simulink model "SpatialKineticsOffline"  (R2013a)
settings: Solver=ode4  StartTime=0.0  StopTime=tf  FixedStep=.001  RelTol=1e-3
PreLoadFcn:
  | load DarkLowerCoeffs
  | load DarkMiddleCoeffs
  | load DarkUpperCoeffs
  | load breaks
values from neighbouring files (symbols this model uses):
  alpha = [ -2.61*pcm -0.53*pcm ]    [SpatialKineticsOpenSourceMain.m]
  breaks = DarkLowerBreaks    [SpatialKineticsOpenSourceMain.m]
  BRIO = 4.266e7    (= 42660000)    [SpatialKineticsOpenSourceMain.m]
  cpc = 2414    [SpatialKineticsOpenSourceMain.m]
  cpp = 2414    [SpatialKineticsOpenSourceMain.m]
  DarkLowerCoeffs = ppDarkLower.coefs    [SpatialKineticsOpenSourceMain.m]
  DarkMiddleCoeffs = ppDarkMiddle.coefs    [SpatialKineticsOpenSourceMain.m]
  DarkRodWorthInserted = -5*Beta    (= -0.00815)    [SpatialKineticsOpenSourceMain.m]
  DarkUpperCoeffs = ppDarkUpper.coefs    [SpatialKineticsOpenSourceMain.m]
  downcomerTimeConstant = 5    [SpatialKineticsOpenSourceMain.m]
  downIO = 216.6*ones(1,3)    [SpatialKineticsOpenSourceMain.m]
  Kc1 = 1/(rho_secondary*V_secondary)    (= 0.00032726218348)    [SpatialKineticsOpenSourceMain.m]
  Kc2 = (h_secondary*A)/(cps*rho_secondary*V_secondary)    (= 1.23242359038)    [SpatialKineticsOpenSourceMain.m]
  Kh1 = 1/(rho_primary*V_primary)    (= 0.000447917898441)    [SpatialKineticsOpenSourceMain.m]
  Kh2 = (h_primary*A)/(cpp*rho_primary*V_primary)    (= 1.29038206968)    [SpatialKineticsOpenSourceMain.m]
  Kw1 = h_primary    (= 23800)    [SpatialKineticsOpenSourceMain.m]
  Kw2 = h_secondary    (= 24500)    [SpatialKineticsOpenSourceMain.m]
  Kw3 = A/(rho_tube*cpw*V_tube)    (= 0.000122049789882)    [SpatialKineticsOpenSourceMain.m]
  PHX_IO = [649.8 637.9 643.7]    [SpatialKineticsOpenSourceMain.m]
  PHX_PI_IO = 271.8    [SpatialKineticsOpenSourceMain.m]
  rate_pct = rate/100    [SpatialKineticsOfflineMain.m]
  rcp_activatetime = 20    [SpatialKineticsOpenSourceMain.m]
  rcpt = 0.1    [SpatialKineticsOpenSourceMain.m]
  reactor_PI_IO = 0.8574    [SpatialKineticsOpenSourceMain.m]
  SVIO = zeros(1,17)    [SpatialKineticsOpenSourceMain.m]
  Ts = 0.001    [SpatialKineticsOpenSourceMain.m]
  xfc0 = -Atemp\btemp*u0    [SpatialKineticsOpenSourceMain.m]
  zone1_IO = [1.041 0.01764 0.04848]    [SpatialKineticsOpenSourceMain.m]
  zone1_thermal_IO = [1044 658.3]    [SpatialKineticsOpenSourceMain.m]
  zone2_IO = [1.098 0.0186 0.05114]    [SpatialKineticsOpenSourceMain.m]
  zone2_thermal_IO = [1083 675.9]    [SpatialKineticsOpenSourceMain.m]
  zone3_IO = [0.9147 0.01549 0.04259]    [SpatialKineticsOpenSourceMain.m]
  zone3_thermal_IO = [1031 692.5]    [SpatialKineticsOpenSourceMain.m]
libraries: simulink x36
(part 3 of 5)

== system SpatialKineticsOffline/RX #2/Parasitic Heat Loss Resulting from DRACS HXs2 ==
  "T_hot " : Inport
  T_cold : Inport  Port=2
  Primary Mass Flow Rate : Inport  Port=3
  MATLAB Function : MATLAB Function  TreatAsAtomicUnit=on
  Specific heat capacity of primary coolant : Constant  Value=cpp
  Total Power Out : Outport
  Power Lost : Outport  Port=2
  Hot Leg Reduction : Outport  Port=3
  wires:
  MATLAB Function/3(Th_red) -> Hot Leg Reduction/1
  MATLAB Function/2(Ploss_MW) -> Power Lost/1
  MATLAB Function/1(P_MW) -> Total Power Out/1
  "T_hot "/1 -> MATLAB Function/1(T_hot)
  T_cold/1 -> MATLAB Function/2(T_cold)
  Primary Mass Flow Rate/1 -> MATLAB Function/3(mdoth)
  Specific heat capacity of primary coolant/1 -> MATLAB Function/4(cpp)

== system SpatialKineticsOffline/RX #2/Primary Heat Exchanger Lumped Model #4 ==
  Primary mass flow  in : Inport
  Primary temp in : Inport  Port=2
  Secondary temp in : Inport  Port=3
  Secondary mass flow in : Inport  Port=4
  Constant : Constant  Value=Kh1  SampleTime=Ts
  Constant1 : Constant  Value=Kh2  SampleTime=Ts
  Constant2 : Constant  Value=Kc1  SampleTime=Ts
  Constant3 : Constant  Value=Kc2  SampleTime=Ts
  Constant4 : Constant  Value=Kw1  SampleTime=Ts
  Constant5 : Constant  Value=Kw2  SampleTime=Ts
  Constant6 : Constant  Value=Kw3  SampleTime=Ts
  Constant7 : Constant  Value=cpp  SampleTime=Ts
  Demux : Demux  Outputs=3
  Display : Display
  Integrator : Integrator  InitialCondition=PHX_IO
  MATLAB Function : MATLAB Function  TreatAsAtomicUnit=on
  Mux2 : Mux  Inputs=7
  Product : Product
  Product1 : Product
  Sum : Sum  Inputs=|+-
  Terminator : Terminator
  W to MW : Gain  Gain=1e-6
  PHx1_Tho : Outport
  PHx1_Tco : Outport  Port=2
  PHx1_HXout : Outport  Port=3
  wires:
  Constant/1 -> Mux2/1
  Constant1/1 -> Mux2/2
  Constant2/1 -> Mux2/3
  Constant3/1 -> Mux2/4
  Constant4/1 -> Mux2/5
  Constant5/1 -> Mux2/6
  Constant6/1 -> Mux2/7
  Mux2/1 -> [PHXpar]
  MATLAB Function/1(dx) -> Integrator/1
  [PHXpar] -> MATLAB Function/6(hxpar)
  Primary temp in/1 -> [Thi], MATLAB Function/2(Thi_input)
  Secondary temp in/1 -> MATLAB Function/3(Tci_input)
  Secondary mass flow in/1 -> MATLAB Function/5(mdotc_input)
  Primary mass flow  in/1 -> [mdoth], MATLAB Function/4(mdoth_input)
  Integrator/1 -> Display/1, Demux/1, MATLAB Function/1(x)
  Demux/3 -> Terminator/1
  Demux/2 -> PHx1_Tco/1
  Demux/1 -> [Tho], PHx1_Tho/1
  Constant7/1 -> Product/2
  [mdoth] -> Product/1
  [Thi] -> Sum/1
  [Tho] -> Sum/2
  Product/1 -> Product1/1
  Sum/1 -> Product1/2
  Product1/1 -> W to MW/1
  W to MW/1 -> PHx1_HXout/1

== system SpatialKineticsOffline/RX #2/Primary Heat Exchanger Lumped Model #5 ==
  Primary mass flow  in : Inport
  Primary temp in : Inport  Port=2
  Secondary temp in : Inport  Port=3
  Secondary mass flow in : Inport  Port=4
  Constant : Constant  Value=Kh1  SampleTime=Ts
  Constant1 : Constant  Value=Kh2  SampleTime=Ts
  Constant2 : Constant  Value=Kc1  SampleTime=Ts
  Constant3 : Constant  Value=Kc2  SampleTime=Ts
  Constant4 : Constant  Value=Kw1  SampleTime=Ts
  Constant5 : Constant  Value=Kw2  SampleTime=Ts
  Constant6 : Constant  Value=Kw3  SampleTime=Ts
  Constant7 : Constant  Value=cpp  SampleTime=Ts
  Demux : Demux  Outputs=3
  Display : Display
  Integrator : Integrator  InitialCondition=PHX_IO
  MATLAB Function : MATLAB Function  TreatAsAtomicUnit=on
  Mux2 : Mux  Inputs=7
  Product : Product
  Product1 : Product
  Sum : Sum  Inputs=|+-
  Terminator : Terminator
  W to MW : Gain  Gain=1e-6
  PHx1_Tho : Outport
  PHx1_Tco : Outport  Port=2
  PHx1_HXout : Outport  Port=3
  wires:
  Constant/1 -> Mux2/1
  Constant1/1 -> Mux2/2
  Constant2/1 -> Mux2/3
  Constant3/1 -> Mux2/4
  Constant4/1 -> Mux2/5
  Constant5/1 -> Mux2/6
  Constant6/1 -> Mux2/7
  Mux2/1 -> [PHXpar]
  MATLAB Function/1(dx) -> Integrator/1
  [PHXpar] -> MATLAB Function/6(hxpar)
  Primary temp in/1 -> [Thi], MATLAB Function/2(Thi_input)
  Secondary temp in/1 -> MATLAB Function/3(Tci_input)
  Secondary mass flow in/1 -> MATLAB Function/5(mdotc_input)
  Primary mass flow  in/1 -> [mdoth], MATLAB Function/4(mdoth_input)
  Integrator/1 -> Display/1, Demux/1, MATLAB Function/1(x)
  Demux/3 -> Terminator/1
  Demux/2 -> PHx1_Tco/1
  Demux/1 -> [Tho], PHx1_Tho/1
  Constant7/1 -> Product/2
  [mdoth] -> Product/1
  [Thi] -> Sum/1
  [Tho] -> Sum/2
  Product/1 -> Product1/1
  Sum/1 -> Product1/2
  Product1/1 -> W to MW/1
  W to MW/1 -> PHx1_HXout/1

== system SpatialKineticsOffline/RX #2/Primary Heat Exchanger Lumped Model #6 ==
  Primary mass flow  in : Inport
  Primary temp in : Inport  Port=2
  Secondary temp in : Inport  Port=3
  Secondary mass flow in : Inport  Port=4
  Constant : Constant  Value=Kh1  SampleTime=Ts
  Constant1 : Constant  Value=Kh2  SampleTime=Ts
  Constant2 : Constant  Value=Kc1  SampleTime=Ts
  Constant3 : Constant  Value=Kc2  SampleTime=Ts
  Constant4 : Constant  Value=Kw1  SampleTime=Ts
  Constant5 : Constant  Value=Kw2  SampleTime=Ts
  Constant6 : Constant  Value=Kw3  SampleTime=Ts
  Constant7 : Constant  Value=cpp  SampleTime=Ts
  Demux : Demux  Outputs=3
  Display : Display
  Integrator : Integrator  InitialCondition=PHX_IO
  MATLAB Function : MATLAB Function  TreatAsAtomicUnit=on
  Mux2 : Mux  Inputs=7
  Product : Product
  Product1 : Product
  Sum : Sum  Inputs=|+-
  Terminator : Terminator
  W to MW : Gain  Gain=1e-6
  PHx1_Tho : Outport
  PHx1_Tco : Outport  Port=2
  PHx1_HXout : Outport  Port=3
  wires:
  Constant7/1 -> Product/2
  [mdoth] -> Product/1
  [Thi] -> Sum/1
  [Tho] -> Sum/2
  Product/1 -> Product1/1
  Sum/1 -> Product1/2
  Product1/1 -> W to MW/1
  W to MW/1 -> PHx1_HXout/1
  Constant/1 -> Mux2/1
  Constant1/1 -> Mux2/2
  Constant2/1 -> Mux2/3
  Constant3/1 -> Mux2/4
  Constant4/1 -> Mux2/5
  Constant5/1 -> Mux2/6
  Constant6/1 -> Mux2/7
  Mux2/1 -> [PHXpar]
  MATLAB Function/1(dx) -> Integrator/1
  [PHXpar] -> MATLAB Function/6(hxpar)
  Primary temp in/1 -> [Thi], MATLAB Function/2(Thi_input)
  Secondary temp in/1 -> MATLAB Function/3(Tci_input)
  Secondary mass flow in/1 -> MATLAB Function/5(mdotc_input)
  Primary mass flow  in/1 -> [mdoth], MATLAB Function/4(mdoth_input)
  Integrator/1 -> Display/1, Demux/1, MATLAB Function/1(x)
  Demux/3 -> Terminator/1
  Demux/2 -> PHx1_Tco/1
  Demux/1 -> [Tho], PHx1_Tho/1

== system SpatialKineticsOffline/RX #2/Ramp Power1 ==
  Max Demand : Inport
  Add : Sum
  Clock : Clock
  Ramp : simulink/Sources/Ramp  slope=rate_pct*42/60  start=tf/2  X0=-rate_pct*42/60*tf/2
  Ramp1 : simulink/Sources/Ramp  slope=-rate_pct*42/60  start=0  X0=0
  Switch : Switch  Threshold=tf/2
  Current Demand : Outport
  wires:
  Switch/1 -> Add/2
  Clock/1 -> Switch/2
  Ramp1/1 -> Switch/3
  Ramp/1 -> Switch/1
  Add/1 -> Current Demand/1
  Max Demand/1 -> Add/1

== system SpatialKineticsOffline/RX #2/Ramp Power2 ==
  Max Demand : Inport
  Add : Sum
  Clock : Clock
  Ramp : simulink/Sources/Ramp  slope=rate_pct*42/60  start=tf/2  X0=-rate_pct*42/60*tf/2
  Ramp1 : simulink/Sources/Ramp  slope=-rate_pct*42/60  start=0  X0=0
  Switch : Switch  Threshold=tf/2
  Current Demand : Outport
  wires:
  Switch/1 -> Add/2
  Clock/1 -> Switch/2
  Ramp1/1 -> Switch/3
  Ramp/1 -> Switch/1
  Add/1 -> Current Demand/1
  Max Demand/1 -> Add/1

== system SpatialKineticsOffline/RX #2/Ramp Power3 ==
  Max Demand : Inport
  Add : Sum
  Clock : Clock
  Ramp : simulink/Sources/Ramp  slope=rate_pct*42/60  start=tf/2  X0=-rate_pct*42/60*tf/2
  Ramp1 : simulink/Sources/Ramp  slope=-rate_pct*42/60  start=0  X0=0
  Switch : Switch  Threshold=tf/2
  Current Demand : Outport
  wires:
  Switch/1 -> Add/2
  Clock/1 -> Switch/2
  Ramp1/1 -> Switch/3
  Ramp/1 -> Switch/1
  Add/1 -> Current Demand/1
  Max Demand/1 -> Add/1

== system SpatialKineticsOffline/RX #2/Reactor Outlet Temperature PI Controller1 ==
  In1 : Inport
  Display : Display
  Display1 : Display
  Display2 : Display
  Gain2 : Gain  Gain=0.01
  Gain5 : Gain  Gain=100
  Integrator : Integrator  InitialCondition=reactor_PI_IO
  Kp : Gain  Gain=.01
  Saturation : Saturate  UpperLimit=1  LowerLimit=0
  Sum12 : Sum  Inputs=+-|
  Sum13 : Sum  Inputs=|+-
  Sum2 : Sum  Inputs=|++
  Out1 : Outport
  wires:
  In1/1 -> Kp/1, Sum13/1
  Sum2/1 -> Display/1, Sum12/1, Saturation/1
  Gain2/1 -> Integrator/1
  Integrator/1 -> Display2/1, Sum2/2
  Kp/1 -> Display1/1, Sum2/1
  Saturation/1 -> Sum12/2, Out1/1
  Sum12/1 -> Gain5/1
  Sum13/1 -> Gain2/1
  Gain5/1 -> Sum13/2

== system SpatialKineticsOffline/RX #2/Secondary-side RCP Dynamics #4 ==
  In1 : Inport
  Digital Clock #1 : DigitalClock  SampleTime=Ts
  RCP #1 : TransferFcn  Numerator=[rcpt]  Denominator=[1 rcpt]
  RCP Dynamics Switch #1 : Switch  Threshold=rcp_activatetime
  Out1 : Outport
  wires:
  In1/1 -> RCP #1/1, RCP Dynamics Switch #1/3
  Digital Clock #1/1 -> RCP Dynamics Switch #1/2
  RCP #1/1 -> RCP Dynamics Switch #1/1
  RCP Dynamics Switch #1/1 -> Out1/1

== system SpatialKineticsOffline/RX #2/Secondary-side RCP Dynamics #5 ==
  In1 : Inport
  Digital Clock#2 : DigitalClock  SampleTime=Ts
  RCP #2 : TransferFcn  Numerator=[rcpt]  Denominator=[1 rcpt]
  RCP Dynamics Switch #2 : Switch  Threshold=rcp_activatetime
  Out1 : Outport
  wires:
  RCP Dynamics Switch #2/1 -> Out1/1
  In1/1 -> RCP #2/1, RCP Dynamics Switch #2/3
  Digital Clock#2/1 -> RCP Dynamics Switch #2/2
  RCP #2/1 -> RCP Dynamics Switch #2/1

== system SpatialKineticsOffline/RX #2/Secondary-side RCP Dynamics #6 ==
  In1 : Inport
  Digital Clock #3 : DigitalClock  SampleTime=Ts
  RCP #3 : TransferFcn  Numerator=[rcpt]  Denominator=[1 rcpt]
  RCP Dynamics Switch #3 : Switch  Threshold=rcp_activatetime
  Out1 : Outport
  wires:
  RCP #3/1 -> RCP Dynamics Switch #3/1
  Digital Clock #3/1 -> RCP Dynamics Switch #3/2
  In1/1 -> RCP #3/1, RCP Dynamics Switch #3/3
  RCP Dynamics Switch #3/1 -> Out1/1

== system SpatialKineticsOffline/RX #3/Downcomer mixing dynamics ==
  PHX Primary Flow 1 : Inport
  PHX Primary Flow 2 : Inport  Port=2
  PHX Primary Flow 3 : Inport  Port=3
  PHX Primary Temp 1 : Inport  Port=4
  PHX Primary Temp 2 : Inport  Port=5
  PHX Primary Temp 3 : Inport  Port=6
  Constant5 : Constant  Value=[0,downcomerTimeConstant]
  Display : Display
  Integrator : Integrator  InitialCondition=downIO
  MATLAB Function1 : MATLAB Function  TreatAsAtomicUnit=on
  Primary Mass Flow Rate : Outport
  Temperature to Reactor T-H : Outport  Port=2
  wires:
  PHX Primary Flow 1/1 -> MATLAB Function1/1(m1)
  PHX Primary Flow 2/1 -> MATLAB Function1/2(m2)
  PHX Primary Flow 3/1 -> MATLAB Function1/3(m3)
  PHX Primary Temp 1/1 -> MATLAB Function1/4(t1)
  PHX Primary Temp 2/1 -> MATLAB Function1/5(t2)
  PHX Primary Temp 3/1 -> MATLAB Function1/6(t3)
  MATLAB Function1/3(xdot) -> Integrator/1
  Integrator/1 -> Display/1, MATLAB Function1/8(x)
  MATLAB Function1/1(y) -> Temperature to Reactor T-H/1
  Constant5/1 -> MATLAB Function1/7(constants)
  MATLAB Function1/2(mtotal) -> Primary Mass Flow Rate/1

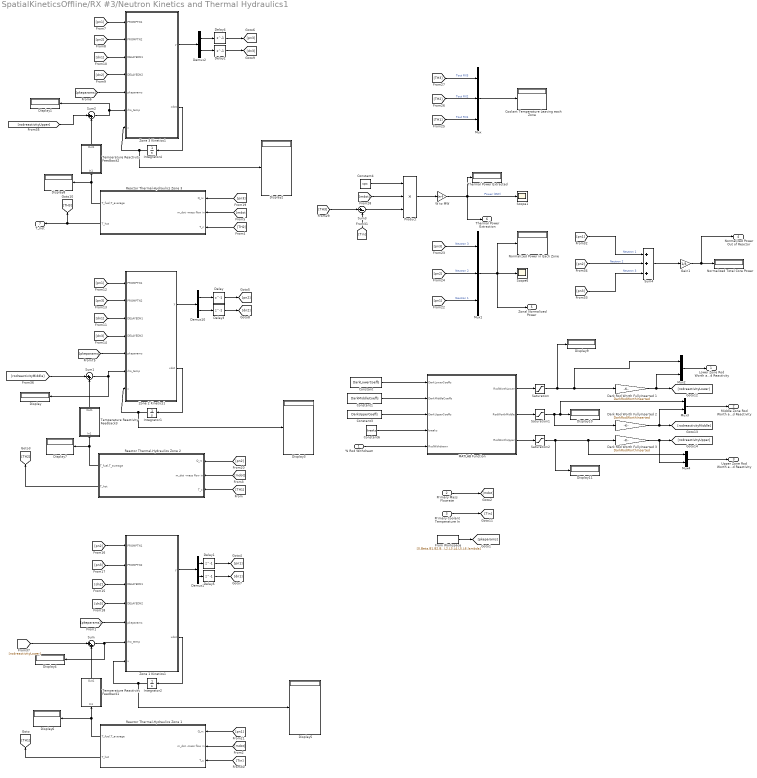
== system SpatialKineticsOffline/RX #3/Neutron Kinetics and Thermal Hydraulics1 ==
  % Rod Withdrawn : Inport
  Primary Mass Flowrate : Inport  Port=2
  Primary Coolant Temperature In : Inport  Port=3
  Constant : Constant  Value=DarkLowerCoeffs
  Constant1 : Constant  Value=DarkMiddleCoeffs
  Constant3 : Constant  Value=DarkUpperCoeffs
  Constant4 : Constant  Value=cpc
  Constant6 : Constant  Value=breaks
  Coolant Temperature Leaving each Zone : Display
  Dark Rod Worth FullyInserted 1 : Gain  Gain=DarkRodWorthInserted
  Dark Rod Worth FullyInserted 2 : Gain  Gain=DarkRodWorthInserted
  Dark Rod Worth FullyInserted 3 : Gain  Gain=DarkRodWorthInserted
  Delay{,1..5} (6 alike) : Delay  DelayLength=1  InitialCondition=0
  Demux1 : Demux  Outputs=2
  Demux10 : Demux  Outputs=2
  Demux2 : Demux  Outputs=2
  Display{,1..11} (12 alike) : Display
  From Workspace : FromWorkspace  VariableName=[0,Beta,B1,B2,B3,B4,B5,B6,L1,L2,L3,L4,L5,L6,lambda]  SampleTime=0
  Gain1 : Gain  Gain=1/3
  Integrator1 : Integrator  InitialCondition=zone2_IO
  Integrator2 : Integrator  InitialCondition=zone1_IO
  Integrator4 : Integrator  InitialCondition=zone3_IO
  MATLAB Function : MATLAB Function  TreatAsAtomicUnit=on
  Mux : Mux  Inputs=3
  Mux1 : Mux  Inputs=3
  Mux2 : Mux  Inputs=2
  Mux3 : Mux  Inputs=2
  Mux4 : Mux  Inputs=2
  Normalized Power in Each Zone : Display
  Normalized Total Core Power : Display
  Product : Product  Inputs=3
  Reactor Thermal-Hydraulics Zone 1 : Subsystem
  Reactor Thermal-Hydraulics Zone 2 : Subsystem
  Reactor Thermal-Hydraulics Zone 3 : Subsystem
  Saturation : Saturate  UpperLimit=inf  LowerLimit=0
  Saturation1 : Saturate  UpperLimit=inf  LowerLimit=0
  Saturation2 : Saturate  UpperLimit=inf  LowerLimit=0
  Scope1 : Scope
      settings: SaveName=ScopeData15
  Scope6 : Scope
      settings: SaveName=ScopeData14
  Sum : Sum  Inputs=|++
  Sum1 : Sum  Inputs=|++
  Sum2 : Sum  Inputs=|++
  Sum3 : Sum  Inputs=|+-
  Sum4 : Sum  Inputs=+++
  Temperature Reactivity Feedback1 : Subsystem
  Temperature Reactivity Feedback2 : Subsystem
  Temperature Reactivity Feedback3 : Subsystem
  Thermal Power Extracted : Display
  W to MW : Gain  Gain=1e-6
  Zone 1 Kinetics1 : MATLAB Function  TreatAsAtomicUnit=on
  Zone 2 Kinetics1 : MATLAB Function  TreatAsAtomicUnit=on
  Zone 3 Kinetics1 : MATLAB Function  TreatAsAtomicUnit=on
  Lower Zone Rod Worth and Reactivity : Outport
  Middle Zone Rod Worth and Reactivity : Outport  Port=2
  Upper Zone Rod Worth and Reactivity : Outport  Port=3
  Normalized Power Out of Reactor : Outport  Port=4
  Zonal Normalized Power : Outport  Port=5
  Thermal Power Extraction : Outport  Port=6
  T_hot : Outport  Port=7
  wires:
  [pkeparams] -> Zone 2 Kinetics1/5(pkeparams)
  Demux1/2 -> Delay5/1
  From Workspace/1 -> [pkeparams]
  Reactor Thermal-Hydraulics Zone 2/1(T_fuel,T_average) -> Display7/1, Temperature Reactivity Feedback3/1(In1)
  [TH1] -> Reactor Thermal-Hydraulics Zone 2/3(T_c)
  Temperature Reactivity Feedback3/1(Out1) -> Sum1/2
  [pkeparams] -> Zone 1 Kinetics1/5(pkeparams)
  Zone 1 Kinetics1/1(y) -> Demux1/1
  Reactor Thermal-Hydraulics Zone 1/1(T_fuel,T_average) -> Temperature Reactivity Feedback1/1(In1), Display6/1
  Temperature Reactivity Feedback1/1(Out1) -> Sum/2
  Demux1/1 -> Delay1/1
  Sum/1 -> Zone 1 Kinetics1/6(rho_temp), Display4/1
  [rodreactivityLower] -> Sum/1
  Sum1/1 -> Zone 2 Kinetics1/6(rho_temp), Display/1
  [rodreactivityMiddle] -> Sum1/1
  Mux/1 -> Coolant Temperature Leaving each Zone/1
  Reactor Thermal-Hydraulics Zone 1/2(T_hot) -> [TH1]
  [mdot] -> Reactor Thermal-Hydraulics Zone 2/2(m_dot -mass flow in)
  [mdot] -> Reactor Thermal-Hydraulics Zone 1/2(m_dot -mass flow in)
  Reactor Thermal-Hydraulics Zone 3/1(T_fuel,T_average) -> Display8/1, Temperature Reactivity Feedback2/1(In1)
  [TH2] -> Reactor Thermal-Hydraulics Zone 3/3(T_c)
  Reactor Thermal-Hydraulics Zone 3/2(T_hot) -> T_hot/1, [TH3]
  Temperature Reactivity Feedback2/1(Out1) -> Sum2/2
  Demux2/1 -> Delay4/1
  Sum2/1 -> Zone 3 Kinetics1/6(rho_temp), Display1/1
  [mdot] -> Reactor Thermal-Hydraulics Zone 3/2(m_dot -mass flow in)
  Delay5/1 -> [dn1]
  Demux2/2 -> Delay2/1
  Reactor Thermal-Hydraulics Zone 2/2(T_hot) -> [TH2]
  Demux10/1 -> Delay/1
  Demux10/2 -> Delay3/1
  Delay4/1 -> [pn3]
  Delay/1 -> [pn2]
  Delay1/1 -> [pn1]
  Delay3/1 -> [dn2]
  Delay2/1 -> [dn3]
  [rodreactivityUpper] -> Sum2/1
  [pn1] -> Zone 2 Kinetics1/1(PROMPTN1)
  [pn3] -> Zone 2 Kinetics1/2(PROMPTN2)
  [dn3] -> Zone 2 Kinetics1/4(DELAYEDN2)
  [dn1] -> Zone 2 Kinetics1/3(DELAYEDN1)
  [pn2] -> Zone 1 Kinetics1/1(PROMPTN1)
  [pn3] -> Zone 1 Kinetics1/2(PROMPTN2)
  [dn2] -> Zone 1 Kinetics1/3(DELAYEDN1)
  [dn3] -> Zone 1 Kinetics1/4(DELAYEDN2)
  [pn3] -> Reactor Thermal-Hydraulics Zone 3/1(Q_rx)
  [pn2] -> Reactor Thermal-Hydraulics Zone 2/1(Q_rx)
  [pn1] -> Reactor Thermal-Hydraulics Zone 1/1(Q_rx)
  Mux1/1 -> Scope6/1, Zonal Normalized Power/1, Normalized Power in Each Zone/1
  [pn1] -> Mux1/3  "Neutron 1"
  [pn3] -> Mux1/1  "Neutron 3"
  [pn2] -> Mux1/2  "Neutron 2"
  [TH1] -> Mux/3  "Tout RX1"
  [TH2] -> Mux/2  "Tout RX2"
  [TH3] -> Mux/1  "Tout RX3"
  Constant4/1 -> Product/1
  [mdot] -> Product/2
  Sum3/1 -> Product/3
  [TH3] -> Sum3/1
  [Tin] -> Reactor Thermal-Hydraulics Zone 1/3(T_c)
  [Tin] -> Sum3/2
  Product/1 -> W to MW/1
  W to MW/1 -> Scope1/1, Thermal Power Extraction/1, Thermal Power Extracted/1  "Power (MW)"
  [pn1] -> Sum4/1  "Neutron 1"
  [pn3] -> Sum4/3  "Neutron 3"
  [pn2] -> Sum4/2  "Neutron 2"
  Sum4/1 -> Gain1/1
  Gain1/1 -> Normalized Power Out of Reactor/1, Normalized Total Core Power/1
  Constant6/1 -> MATLAB Function/4(breaks)
  Constant3/1 -> MATLAB Function/3(DarkUpperCoeffs)
  Constant1/1 -> MATLAB Function/2(DarkMiddleCoeffs)
  Constant/1 -> MATLAB Function/1(DarkLowerCoeffs)
  MATLAB Function/1(RodWorthLower) -> Saturation/1
  MATLAB Function/2(RodWorthMiddle) -> Saturation1/1
  MATLAB Function/3(RodWorthUpper) -> Saturation2/1
  % Rod Withdrawn/1 -> MATLAB Function/5(RodWithdrawn)
  Saturation/1 -> Mux2/1, Dark Rod Worth FullyInserted 1/1, Display9/1
  Saturation1/1 -> Dark Rod Worth FullyInserted 2/1, Mux3/1, Display10/1
  Saturation2/1 -> Mux4/1, Dark Rod Worth FullyInserted 3/1, Display11/1
  Dark Rod Worth FullyInserted 1/1 -> Mux2/2, [rodreactivityLower]
  Dark Rod Worth FullyInserted 2/1 -> Mux3/2, [rodreactivityMiddle]
  Dark Rod Worth FullyInserted 3/1 -> Mux4/2, [rodreactivityUpper]
  Primary Mass Flowrate/1 -> [mdot]
  Primary Coolant Temperature In/1 -> [Tin]
  Mux2/1 -> Lower Zone Rod Worth and Reactivity/1
  Mux3/1 -> Middle Zone Rod Worth and Reactivity/1
  Mux4/1 -> Upper Zone Rod Worth and Reactivity/1
  Integrator4/1 -> Zone 3 Kinetics1/7(x), Display2/1
  Zone 3 Kinetics1/2(xdot) -> Integrator4/1
  [pkeparams] -> Zone 3 Kinetics1/5(pkeparams)
  [dn2] -> Zone 3 Kinetics1/4(DELAYEDN2)
  [dn1] -> Zone 3 Kinetics1/3(DELAYEDN1)
  [pn2] -> Zone 3 Kinetics1/2(PROMPTN2)
  [pn1] -> Zone 3 Kinetics1/1(PROMPTN1)
  Zone 3 Kinetics1/1(y) -> Demux2/1
  Zone 2 Kinetics1/2(xdot) -> Integrator1/1
  Integrator1/1 -> Zone 2 Kinetics1/7(x), Display3/1
  Zone 2 Kinetics1/1(y) -> Demux10/1
  Zone 1 Kinetics1/2(xdot) -> Integrator2/1
  Integrator2/1 -> Display5/1, Zone 1 Kinetics1/7(x)

== system SpatialKineticsOffline/RX #3/PI Controller with Integral Anti-windup for HX4 ==
  HX Power Produced : Inport
  Power Setpoint : Inport  Port=2
  Cold_flow_high5 : Constant  Value=370
  Cold_flow_low2 : Constant  Value=0
  Display : Display
  Gain5 : Gain  Gain=15
  Integrator2 : Integrator  InitialCondition=PHX_PI_IO
  Ki2 : Gain  Gain=0.14145998
  Kp2 : Gain  Gain=1.083074
  Saturation Dynamic2 : simulink/Discontinuities/Saturation Dynamic  OutMin=[]  OutMax=[]  OutDataTypeStr=Inherit: Same as second input  OutDataType=fixdt(1, 16)  OutScaling=2^-10  DoSatur=off
  Sum12 : Sum  Inputs=+-|
  Sum13 : Sum  Inputs=|+-
  Sum14 : Sum  Inputs=|+-
  Sum15 : Sum  Inputs=|++
  Control Action : Outport
  wires:
  HX Power Produced/1 -> Sum14/2
  Cold_flow_low2/1 -> Saturation Dynamic2/3
  Cold_flow_high5/1 -> Saturation Dynamic2/1
  Sum14/1 -> Kp2/1, Sum13/1
  Power Setpoint/1 -> Sum14/1
  Sum12/1 -> Gain5/1
  Integrator2/1 -> Display/1, Sum15/2
  Gain5/1 -> Sum13/2
  Sum13/1 -> Ki2/1
  Ki2/1 -> Integrator2/1
  Kp2/1 -> Sum15/1
  Saturation Dynamic2/1 -> Control Action/1, Sum12/2
  Sum15/1 -> Saturation Dynamic2/2, Sum12/1

== system SpatialKineticsOffline/RX #3/PI Controller with Integral Anti-windup for HX5 ==
  HX Power Produced : Inport
  Power Setpoint : Inport  Port=2
  Cold_flow_high5 : Constant  Value=370
  Cold_flow_low2 : Constant  Value=0
  Display : Display
  Gain5 : Gain  Gain=15
  Integrator2 : Integrator  InitialCondition=PHX_PI_IO
  Ki2 : Gain  Gain=0.14145998
  Kp2 : Gain  Gain=1.083074
  Saturation Dynamic2 : simulink/Discontinuities/Saturation Dynamic  OutMin=[]  OutMax=[]  OutDataTypeStr=Inherit: Same as second input  OutDataType=fixdt(1, 16)  OutScaling=2^-10  DoSatur=off
  Sum12 : Sum  Inputs=+-|
  Sum13 : Sum  Inputs=|+-
  Sum14 : Sum  Inputs=|+-
  Sum15 : Sum  Inputs=|++
  Control Action : Outport
  wires:
  HX Power Produced/1 -> Sum14/2
  Cold_flow_low2/1 -> Saturation Dynamic2/3
  Cold_flow_high5/1 -> Saturation Dynamic2/1
  Sum14/1 -> Kp2/1, Sum13/1
  Power Setpoint/1 -> Sum14/1
  Sum12/1 -> Gain5/1
  Integrator2/1 -> Display/1, Sum15/2
  Gain5/1 -> Sum13/2
  Sum13/1 -> Ki2/1
  Ki2/1 -> Integrator2/1
  Kp2/1 -> Sum15/1
  Saturation Dynamic2/1 -> Control Action/1, Sum12/2
  Sum15/1 -> Saturation Dynamic2/2, Sum12/1

== system SpatialKineticsOffline/RX #3/PI Controller with Integral Anti-windup for HX6 ==
  HX Power Produced : Inport
  Power Setpoint : Inport  Port=2
  Cold_flow_high5 : Constant  Value=370
  Cold_flow_low2 : Constant  Value=0
  Display : Display
  Gain5 : Gain  Gain=15
  Integrator2 : Integrator  InitialCondition=PHX_PI_IO
  Ki2 : Gain  Gain=0.14145998
  Kp2 : Gain  Gain=1.083074
  Saturation Dynamic2 : simulink/Discontinuities/Saturation Dynamic  OutMin=[]  OutMax=[]  OutDataTypeStr=Inherit: Same as second input  OutDataType=fixdt(1, 16)  OutScaling=2^-10  DoSatur=off
  Sum12 : Sum  Inputs=+-|
  Sum13 : Sum  Inputs=|+-
  Sum14 : Sum  Inputs=|+-
  Sum15 : Sum  Inputs=|++
  Control Action : Outport
  wires:
  HX Power Produced/1 -> Sum14/2
  Cold_flow_low2/1 -> Saturation Dynamic2/3
  Cold_flow_high5/1 -> Saturation Dynamic2/1
  Sum14/1 -> Kp2/1, Sum13/1
  Power Setpoint/1 -> Sum14/1
  Sum12/1 -> Gain5/1
  Gain5/1 -> Sum13/2
  Sum13/1 -> Ki2/1
  Ki2/1 -> Integrator2/1
  Kp2/1 -> Sum15/1
  Saturation Dynamic2/1 -> Control Action/1, Sum12/2
  Sum15/1 -> Saturation Dynamic2/2, Sum12/1
  Integrator2/1 -> Display/1, Sum15/2

== system SpatialKineticsOffline/RX #3/Parasitic Heat Loss Resulting from DRACS HXs2 ==
  "T_hot " : Inport
  T_cold : Inport  Port=2
  Primary Mass Flow Rate : Inport  Port=3
  MATLAB Function : MATLAB Function  TreatAsAtomicUnit=on
  Specific heat capacity of primary coolant : Constant  Value=cpp
  Total Power Out : Outport
  Power Lost : Outport  Port=2
  Hot Leg Reduction : Outport  Port=3
  wires:
  MATLAB Function/3(Th_red) -> Hot Leg Reduction/1
  MATLAB Function/2(Ploss_MW) -> Power Lost/1
  MATLAB Function/1(P_MW) -> Total Power Out/1
  "T_hot "/1 -> MATLAB Function/1(T_hot)
  T_cold/1 -> MATLAB Function/2(T_cold)
  Primary Mass Flow Rate/1 -> MATLAB Function/3(mdoth)
  Specific heat capacity of primary coolant/1 -> MATLAB Function/4(cpp)

== system SpatialKineticsOffline/RX #3/Primary Heat Exchanger Lumped Model #4 ==
  Primary mass flow  in : Inport
  Primary temp in : Inport  Port=2
  Secondary temp in : Inport  Port=3
  Secondary mass flow in : Inport  Port=4
  Constant : Constant  Value=Kh1  SampleTime=Ts
  Constant1 : Constant  Value=Kh2  SampleTime=Ts
  Constant2 : Constant  Value=Kc1  SampleTime=Ts
  Constant3 : Constant  Value=Kc2  SampleTime=Ts
  Constant4 : Constant  Value=Kw1  SampleTime=Ts
  Constant5 : Constant  Value=Kw2  SampleTime=Ts
  Constant6 : Constant  Value=Kw3  SampleTime=Ts
  Constant7 : Constant  Value=cpp  SampleTime=Ts
  Demux : Demux  Outputs=3
  Display : Display
  Integrator : Integrator  InitialCondition=PHX_IO
  MATLAB Function : MATLAB Function  TreatAsAtomicUnit=on
  Mux2 : Mux  Inputs=7
  Product : Product
  Product1 : Product
  Sum : Sum  Inputs=|+-
  Terminator : Terminator
  W to MW : Gain  Gain=1e-6
  PHx1_Tho : Outport
  PHx1_Tco : Outport  Port=2
  PHx1_HXout : Outport  Port=3
  wires:
  Constant/1 -> Mux2/1
  Constant1/1 -> Mux2/2
  Constant2/1 -> Mux2/3
  Constant3/1 -> Mux2/4
  Constant4/1 -> Mux2/5
  Constant5/1 -> Mux2/6
  Constant6/1 -> Mux2/7
  Mux2/1 -> [PHXpar]
  MATLAB Function/1(dx) -> Integrator/1
  [PHXpar] -> MATLAB Function/6(hxpar)
  Primary temp in/1 -> [Thi], MATLAB Function/2(Thi_input)
  Secondary temp in/1 -> MATLAB Function/3(Tci_input)
  Secondary mass flow in/1 -> MATLAB Function/5(mdotc_input)
  Primary mass flow  in/1 -> [mdoth], MATLAB Function/4(mdoth_input)
  Integrator/1 -> Display/1, Demux/1, MATLAB Function/1(x)
  Demux/3 -> Terminator/1
  Demux/2 -> PHx1_Tco/1
  Demux/1 -> [Tho], PHx1_Tho/1
  Constant7/1 -> Product/2
  [mdoth] -> Product/1
  [Thi] -> Sum/1
  [Tho] -> Sum/2
  Product/1 -> Product1/1
  Sum/1 -> Product1/2
  Product1/1 -> W to MW/1
  W to MW/1 -> PHx1_HXout/1

== matlab function SpatialKineticsOffline/RX #1/Neutron Kinetics and Thermal Hydraulics/Zone 2 Kinetics1 ==
  data: PROMPTN1 input; PROMPTN2 input; DELAYEDN1 input; DELAYEDN2 input; pkeparams input; rho_temp input; x input; y output; xdot output
function [y,xdot] = Zone2Kinetics(PROMPTN1,PROMPTN2,DELAYEDN1,DELAYEDN2,pkeparams,rho_temp,x)
%#codegen
% 
% %Unpackage the prompt and delayed neutron sources
% 
% %Prompt neuton unpackaging
N1 = PROMPTN1;
N2 = PROMPTN2;

% %Delayed neutron unpackaging
D1 = DELAYEDN1;
D2 = DELAYEDN2;

%PKE parameter load
Beta = pkeparams(1); B1 = pkeparams(2); B2 = pkeparams(3); 
L1 = pkeparams(8); L2 = pkeparams(9); 
lambda = pkeparams(14);

%Reactivity coupling effects from other zones
alpha = (1-Beta)/lambda;
%The numerical values (0.005) included herein represent the
%neutronic coupling coefficients that couple the delayed and prompt
%neutrons to other core regions.  It is quickly seen that these are
%translated into a reactivity.
rho_1 = lambda*0.005*(alpha*(N1/x(1))+0.005*(1/lambda)*D1/x(1));
rho_2 = lambda*0.005*(alpha*(N2/x(1))+0.005*(1/lambda)*D2/x(1));

%Reactor Point Kinetics State Equation
rho_t=rho_temp+rho_1+rho_2;

A = [(rho_t-Beta)/lambda L1/lambda L2/lambda;...
    B1 -L1 0;...
    B2 0 -L2];

C = [1 0 0;...
    0 L1 L2];

% xdot = zeros(3,1,'double');
xdot = A*x;
% y = zeros(2,1,'double');
y = C*x;

return

== matlab function SpatialKineticsOffline/RX #3/MATLAB Function ==
  data: m1 input; SHX_massflow output; m2 input; m3 input; T1 input; T2 input; T3 input; SHX_temp output
function [SHX_massflow,SHX_temp] = SaltVaultMassAveraging(m1,m2,m3,T1,T2,T3)

SHX_massflow=m1+m2+m3;

SHX_temp=(m1/SHX_massflow)*T1+(m2/SHX_massflow)*T2+(m3/SHX_massflow)*T3;

return

== matlab function SpatialKineticsOffline/RX #4/MATLAB Function ==
  data: m1 input; SHX_massflow output; m2 input; m3 input; T1 input; T2 input; T3 input; SHX_temp output
function [SHX_massflow,SHX_temp] = SaltVaultMassAveraging(m1,m2,m3,T1,T2,T3)

SHX_massflow=m1+m2+m3;

SHX_temp=(m1/SHX_massflow)*T1+(m2/SHX_massflow)*T2+(m3/SHX_massflow)*T3;

return

== matlab function SpatialKineticsOffline/Brayton Cycle #1/MATLAB Function ==
  data: y output; Tturb_out output; Tcomp_out output; xdot output; Tcomp_in input; Tturb_in input; mdot input; constants input; x input
function [y,Tturb_out,Tcomp_out,xdot]=BraytonCycle(Tcomp_in,Tturb_in,mdot,constants,x)

eta_comp=constants(1); %compressor efficiency
eta_turb=constants(2); %turbine efficiency
r=constants(3); %isotropic pressure ratio
cpCO2_turb=constants(4); %specific heat capacity of gas (which is air)
cpCO2_comp=constants(5);
% rhoCO2=constants(6);
tau_turb=constants(7); %Compressor-turbine time constant

Tcomp_out=(Tcomp_in+273)*((r-1)/eta_comp+1)-273; %Compressor outlet temperature
Tturb_out=(Tturb_in+273)*(1-eta_turb*(1-(1/r)))-273; %Turbine outlet temperature

Pturb=mdot*cpCO2_turb*(Tturb_in-Tturb_out); %Turbine power
Pcomp=mdot*cpCO2_comp*(Tcomp_out-Tcomp_in); %Compressor power

u=Pturb-Pcomp; %Preliminary input to state space model;

%Our state is the mechanical / shaft power produced 

A=-1/tau_turb; 
B=1/tau_turb;
C=1;
D=0;

%We are calcuating only the net mechanical output power, for now.
xdot=A*x+B*u;
y=C*x+D*u;

return

== matlab function SpatialKineticsOffline/RX #2/Neutron Kinetics and Thermal Hydraulics1/Reactor Thermal-Hydraulics Zone 2/MATLAB Function ==
  data: m_dot input; Q_rx input; constants input; y output; T_c input; x input; x_dot output
function [y,x_dot] =FuelCoolantHX(m_dot,Q_rx,constants,T_c,x)

cpc=constants(1);
cpf=constants(2);
mc=constants(3);
mf=constants(4);
uh=constants(5);
Ar=constants(6);

A=[-(uh*Ar)/(mf*cpf), (uh*Ar)/(mf*cpf); (uh*Ar)/(mc*cpc), -(uh*Ar)/(mc*cpc)-(2*m_dot)/mc];

K=125000000/3;

b=[K/(mf*cpf), 0; 0 2*m_dot/mc];

u=[Q_rx; T_c];

x_dot=A*x+b*u;

C=[1 0; 0 1; 0 2];
D=[0 0;0 0; 0 -1];

y=C*x+D*u;

return

== matlab function SpatialKineticsOffline/RX #2/Neutron Kinetics and Thermal Hydraulics1/Zone 1 Kinetics1 ==
  data: PROMPTN1 input; PROMPTN2 input; DELAYEDN1 input; DELAYEDN2 input; pkeparams input; rho_temp input; x input; y output; xdot output
function [y,xdot] = Zone1Kinetics(PROMPTN1,PROMPTN2,DELAYEDN1,DELAYEDN2,pkeparams,rho_temp,x)
%#codegen
% 
% K=reshape(Lcoupling,12,12); %Reshape the coupling matrix
% 
% %Unpackage the prompt and delayed neutron sources
% 
% %Prompt neuton unpackaging
N1 = PROMPTN1;
N2 = PROMPTN2;
% N2 = PROMPTN(2); N3 = PROMPTN(3); N4 = PROMPTN(4);
% N5 = PROMPTN(5); N6 = PROMPTN(6); N7 = PROMPTN(7);
% N8 = PROMPTN(8); N9 = PROMPTN(9); N10 = PROMPTN(10);
% N11 = PROMPTN(11); N12 = PROMPTN(12);
% 
% %Delayed neutron unpackaging
D1 = DELAYEDN1;
D2 = DELAYEDN2;
% D2 = DELAYEDN(2); D3 = DELAYEDN(3); D4 = DELAYEDN(4);
% D5 = DELAYEDN(5); D6 = DELAYEDN(6); D7 = DELAYEDN(7);
% D8 = DELAYEDN(8); D9 = DELAYEDN(9); D10 = DELAYEDN(10);
% D11 = DELAYEDN(11); D12 = DELAYEDN(12);

%PKE parameter load
Beta = pkeparams(1); B1 = pkeparams(2); B2 = pkeparams(3); B3 = pkeparams(4);
B4 = pkeparams(5); B5 = pkeparams(6); B6 = pkeparams(7); L1 = pkeparams(8);
L2 = pkeparams(9); L3 = pkeparams(10); L4 = pkeparams(11); L5 = pkeparams(12);
L6 = pkeparams(13); lambda = pkeparams(14);

%Reactivity coupling effects from other zones
alpha = (1-Beta)/lambda;
% 
rho_1 = lambda*0.005*(alpha*(N1/x(1))+0.005*(1/lambda)*D1/x(1));
rho_2 = lambda*0.002*(alpha*(N2/x(1))+0.002*(1/lambda)*D2/x(1));
% rho_3 = lambda*K(11,3)*(alpha*(N3/x(1))+(1/lambda)*D3/x(1));
% rho_4 = lambda*K(11,4)*(alpha*(N4/x(1))+(1/lambda)*D4/x(1));
% rho_5 = lambda*K(11,5)*(alpha*(N5/x(1))+(1/lambda)*D5/x(1));
% rho_6 = lambda*K(11,6)*(alpha*(N6/x(1))+(1/lambda)*D6/x(1));
% rho_7 = lambda*K(11,7)*(alpha*(N7/x(1))+(1/lambda)*D7/x(1));
% rho_8 = lambda*K(11,8)*(alpha*(N8/x(1))+(1/lambda)*D8/x(1));
% rho_9 = lambda*K(11,9)*(alpha*(N9/x(1))+(1/lambda)*D9/x(1));
% rho_10 = lambda*K(11,10)*(alpha*(N10/x(1))+(1/lambda)*D10/x(1));
% % rho_11 = lambda*K(11,11)*(alpha*(N11/x(1))+(1/lambda)*D11/x(1));
% rho_12 = lambda*K(11,12)*(alpha*(N12/x(1))+(1/lambda)*D12/x(1));
% 
% %Total reactivity
% 
% rho_t=rho_temp+rho_1+rho_2+rho_3+rho_4+rho_5+rho_6+rho_7+rho_8+rho_9+rho_10+rho_12;

%Reactor Point Kinetics State Equation
rho_t=rho_temp+rho_1+rho_2;

A = [(rho_t-Beta)/lambda L1/lambda L2/lambda;...
    B1 -L1 0;...
    B2 0 -L2];

C = [1 0 0;...
    0 L1 L2];

xdot = zeros(3,1,'double');
xdot = A*x;
y = zeros(2,1,'double');
y = C*x;

return

== matlab function SpatialKineticsOffline/Brayton Cycle #2/MATLAB Function4 ==
  data: y output; Tturb_out output; Tcomp_out output; xdot output; Tcomp_in input; Tturb_in input; mdot input; constants input; x input
function [y,Tturb_out,Tcomp_out,xdot]=BraytonCycle(Tcomp_in,Tturb_in,mdot,constants,x)

eta_comp=constants(1); %compressor efficiency
eta_turb=constants(2); %turbine efficiency
r=constants(3); %isotropic pressure ratio
cpCO2_turb=constants(4); %specific heat capacity of gas (which is air)
cpCO2_comp=constants(5);
% rhoCO2=constants(6);
tau_turb=constants(7); %Compressor-turbine time constant

Tcomp_out=(Tcomp_in+273)*((r-1)/eta_comp+1)-273; %Compressor outlet temperature
Tturb_out=(Tturb_in+273)*(1-eta_turb*(1-(1/r)))-273; %Turbine outlet temperature

Pturb=mdot*cpCO2_turb*(Tturb_in-Tturb_out); %Turbine power
Pcomp=mdot*cpCO2_comp*(Tcomp_out-Tcomp_in); %Compressor power

u=Pturb-Pcomp; %Preliminary input to state space model;

%Our state is the mechanical / shaft power produced 

A=-1/tau_turb; 
B=1/tau_turb;
C=1;
D=0;

%We are calcuating only the net mechanical output power, for now.
xdot=A*x+B*u;
y=C*x+D*u;

return

== matlab function SpatialKineticsOffline/RX #3/Neutron Kinetics and Thermal Hydraulics1/MATLAB Function ==
  data: DarkLowerCoeffs input; RodWorthLower output; DarkMiddleCoeffs input; DarkUpperCoeffs input; breaks input; RodWithdrawn input; RodWorthMiddle output; RodWorthUpper output
function [RodWorthLower,RodWorthMiddle,RodWorthUpper] = RodWorthIAEACurveFit(DarkLowerCoeffs,DarkMiddleCoeffs,DarkUpperCoeffs,breaks,...
    RodWithdrawn)

persistent L M U

for i = 1:length(breaks)-1
    if RodWithdrawn >= breaks(i) && RodWithdrawn < breaks(i+1)
        L = polyval(DarkLowerCoeffs(i,:),RodWithdrawn - breaks(i));
        M = polyval(DarkMiddleCoeffs(i,:),RodWithdrawn - breaks(i));
        U = polyval(DarkUpperCoeffs(i,:),RodWithdrawn - breaks(i));
        RodWorthLower = L;
        RodWorthMiddle = M;
        RodWorthUpper = U;
        return
    else
        L = 0;
        M = 0;
        U = 0;
        continue
    end
end

RodWorthLower = L;
RodWorthMiddle = M;
RodWorthUpper = U;

== matlab function SpatialKineticsOffline/RX #3/Neutron Kinetics and Thermal Hydraulics1/Zone 1 Kinetics1 ==
  data: PROMPTN1 input; PROMPTN2 input; DELAYEDN1 input; DELAYEDN2 input; pkeparams input; rho_temp input; x input; y output; xdot output
function [y,xdot] = Zone1Kinetics(PROMPTN1,PROMPTN2,DELAYEDN1,DELAYEDN2,pkeparams,rho_temp,x)
%#codegen
% 
% K=reshape(Lcoupling,12,12); %Reshape the coupling matrix
% 
% %Unpackage the prompt and delayed neutron sources
% 
% %Prompt neuton unpackaging
N1 = PROMPTN1;
N2 = PROMPTN2;
% N2 = PROMPTN(2); N3 = PROMPTN(3); N4 = PROMPTN(4);
% N5 = PROMPTN(5); N6 = PROMPTN(6); N7 = PROMPTN(7);
% N8 = PROMPTN(8); N9 = PROMPTN(9); N10 = PROMPTN(10);
% N11 = PROMPTN(11); N12 = PROMPTN(12);
% 
% %Delayed neutron unpackaging
D1 = DELAYEDN1;
D2 = DELAYEDN2;
% D2 = DELAYEDN(2); D3 = DELAYEDN(3); D4 = DELAYEDN(4);
% D5 = DELAYEDN(5); D6 = DELAYEDN(6); D7 = DELAYEDN(7);
% D8 = DELAYEDN(8); D9 = DELAYEDN(9); D10 = DELAYEDN(10);
% D11 = DELAYEDN(11); D12 = DELAYEDN(12);

%PKE parameter load
Beta = pkeparams(1); B1 = pkeparams(2); B2 = pkeparams(3); B3 = pkeparams(4);
B4 = pkeparams(5); B5 = pkeparams(6); B6 = pkeparams(7); L1 = pkeparams(8);
L2 = pkeparams(9); L3 = pkeparams(10); L4 = pkeparams(11); L5 = pkeparams(12);
L6 = pkeparams(13); lambda = pkeparams(14);

%Reactivity coupling effects from other zones
alpha = (1-Beta)/lambda;
% 
rho_1 = lambda*0.005*(alpha*(N1/x(1))+0.005*(1/lambda)*D1/x(1));
rho_2 = lambda*0.002*(alpha*(N2/x(1))+0.002*(1/lambda)*D2/x(1));
% rho_3 = lambda*K(11,3)*(alpha*(N3/x(1))+(1/lambda)*D3/x(1));
% rho_4 = lambda*K(11,4)*(alpha*(N4/x(1))+(1/lambda)*D4/x(1));
% rho_5 = lambda*K(11,5)*(alpha*(N5/x(1))+(1/lambda)*D5/x(1));
% rho_6 = lambda*K(11,6)*(alpha*(N6/x(1))+(1/lambda)*D6/x(1));
% rho_7 = lambda*K(11,7)*(alpha*(N7/x(1))+(1/lambda)*D7/x(1));
% rho_8 = lambda*K(11,8)*(alpha*(N8/x(1))+(1/lambda)*D8/x(1));
% rho_9 = lambda*K(11,9)*(alpha*(N9/x(1))+(1/lambda)*D9/x(1));
% rho_10 = lambda*K(11,10)*(alpha*(N10/x(1))+(1/lambda)*D10/x(1));
% % rho_11 = lambda*K(11,11)*(alpha*(N11/x(1))+(1/lambda)*D11/x(1));
% rho_12 = lambda*K(11,12)*(alpha*(N12/x(1))+(1/lambda)*D12/x(1));
% 
% %Total reactivity
% 
% rho_t=rho_temp+rho_1+rho_2+rho_3+rho_4+rho_5+rho_6+rho_7+rho_8+rho_9+rho_10+rho_12;

%Reactor Point Kinetics State Equation
rho_t=rho_temp+rho_1+rho_2;

A = [(rho_t-Beta)/lambda L1/lambda L2/lambda;...
    B1 -L1 0;...
    B2 0 -L2];

C = [1 0 0;...
    0 L1 L2];

xdot = zeros(3,1,'double');
xdot = A*x;
y = zeros(2,1,'double');
y = C*x;

return

== matlab function SpatialKineticsOffline/RX #1/Primary Heat Exchanger Lumped Model #2/MATLAB Function ==
  data: x input; dx output; Thi_input input; Tci_input input; mdoth_input input; mdotc_input input; hxpar input
function dx  = fcn(x,Thi_input,Tci_input,mdoth_input,mdotc_input,hxpar)
%#codegen

%%%%% Temperature inputs
Thi = Thi_input;
Tci = Tci_input;

%%%%% Mass flow rate inputs
mdoth = mdoth_input;
mdotc = mdotc_input;

%%%%%% Parameters
kh1 = hxpar(1);
kh2 = hxpar(2);
kc1 = hxpar(3);
kc2 = hxpar(4);
kw1   = hxpar(5);
kw2   = hxpar(6);
kw3   = hxpar(7);

%%%%% States
%%%%% x = [x1 x2 x3]^T
%%%%% x1 is the hot-leg inlet temp
%%%%% x2 is the cold-leg inlet temp
%%%%% x3 is the wall temp
x1 = x(1);
x2 = x(2);
x3 = x(3);

%%%%% State equation
dx1 = -kh2*(x1-x3) + kh1*mdoth*(Thi-x1);
dx2 = kc2*(x3-x2) + kc1*mdotc*(Tci-x2);
dx3 = kw3*kw1*(x1-x3) - kw3*kw2*(x3-x2);

dx  = [dx1;dx2;dx3];

% %%%%%  Heat Transfer Output in MegaWatts
% HXout = mdoth*cpp*(Thi-x1) * 1e-6; 
% 
% %%%%% outlet Temperatures
% Tho = x(1);
% Tco = x(2);

== matlab function SpatialKineticsOffline/RX #2/Primary Heat Exchanger Lumped Model #5/MATLAB Function ==
  data: x input; dx output; Thi_input input; Tci_input input; mdoth_input input; mdotc_input input; hxpar input
function dx  = fcn(x,Thi_input,Tci_input,mdoth_input,mdotc_input,hxpar)
%#codegen

%%%%% Temperature inputs
Thi = Thi_input;
Tci = Tci_input;

%%%%% Mass flow rate inputs
mdoth = mdoth_input;
mdotc = mdotc_input;

%%%%%% Parameters
kh1 = hxpar(1);
kh2 = hxpar(2);
kc1 = hxpar(3);
kc2 = hxpar(4);
kw1   = hxpar(5);
kw2   = hxpar(6);
kw3   = hxpar(7);


%%%%% States
%%%%% x = [x1 x2 x3]^T
%%%%% x1 is the hot-leg inlet temp
%%%%% x2 is the cold-leg inlet temp
%%%%% x3 is the wall temp
x1 = x(1);
x2 = x(2);
x3 = x(3);

%%%%% State equation
dx1 = -kh2*(x1-x3) + kh1*mdoth*(Thi-x1);
dx2 = kc2*(x3-x2) + kc1*mdotc*(Tci-x2);
dx3 = kw3*kw1*(x1-x3) - kw3*kw2*(x3-x2);

dx  = [dx1;dx2;dx3];

% %%%%%  Heat Transfer Output in MegaWatts
% HXout = mdoth*cpp*(Thi-x1) * 1e-6; 
% 
% %%%%% outlet Temperatures
% Tho = x(1);
% Tco = x(2);

== matlab function SpatialKineticsOffline/RX #4/Neutron Kinetics and Thermal Hydraulics/Reactor Thermal-Hydraulics Zone 2/MATLAB Function ==
  data: m_dot input; Q_rx input; constants input; y output; T_c input; x input; x_dot output
function [y,x_dot] =FuelCoolantHX(m_dot,Q_rx,constants,T_c,x)

cpc=constants(1);
cpf=constants(2);
mc=constants(3);
mf=constants(4);
uh=constants(5);
Ar=constants(6);

A=[-(uh*Ar)/(mf*cpf), (uh*Ar)/(mf*cpf); (uh*Ar)/(mc*cpc), -(uh*Ar)/(mc*cpc)-(2*m_dot)/mc];

K=125000000/3;

b=[K/(mf*cpf), 0; 0 2*m_dot/mc];

u=[Q_rx; T_c];

x_dot=A*x+b*u;

C=[1 0; 0 1; 0 2];
D=[0 0;0 0; 0 -1];

y=C*x+D*u;

return

== matlab function SpatialKineticsOffline/RX #4/Neutron Kinetics and Thermal Hydraulics/Zone 2 Kinetics1 ==
  data: PROMPTN1 input; PROMPTN2 input; DELAYEDN1 input; DELAYEDN2 input; pkeparams input; rho_temp input; x input; y output; xdot output
function [y,xdot] = Zone2Kinetics(PROMPTN1,PROMPTN2,DELAYEDN1,DELAYEDN2,pkeparams,rho_temp,x)
%#codegen
% 
% K=reshape(Lcoupling,12,12); %Reshape the coupling matrix
% 
% %Unpackage the prompt and delayed neutron sources
% 
% %Prompt neuton unpackaging
N1 = PROMPTN1;
N2 = PROMPTN2;
% N2 = PROMPTN(2); N3 = PROMPTN(3); N4 = PROMPTN(4);
% N5 = PROMPTN(5); N6 = PROMPTN(6); N7 = PROMPTN(7);
% N8 = PROMPTN(8); N9 = PROMPTN(9); N10 = PROMPTN(10);
% N11 = PROMPTN(11); N12 = PROMPTN(12);
% 
% %Delayed neutron unpackaging
D1 = DELAYEDN1;
D2 = DELAYEDN2;
% D2 = DELAYEDN(2); D3 = DELAYEDN(3); D4 = DELAYEDN(4);
% D5 = DELAYEDN(5); D6 = DELAYEDN(6); D7 = DELAYEDN(7);
% D8 = DELAYEDN(8); D9 = DELAYEDN(9); D10 = DELAYEDN(10);
% D11 = DELAYEDN(11); D12 = DELAYEDN(12);

%PKE parameter load
Beta = pkeparams(1); B1 = pkeparams(2); B2 = pkeparams(3); B3 = pkeparams(4);
B4 = pkeparams(5); B5 = pkeparams(6); B6 = pkeparams(7); L1 = pkeparams(8);
L2 = pkeparams(9); L3 = pkeparams(10); L4 = pkeparams(11); L5 = pkeparams(12);
L6 = pkeparams(13); lambda = pkeparams(14);

%Reactivity coupling effects from other zones
alpha = (1-Beta)/lambda;
% 
rho_1 = lambda*0.005*(alpha*(N1/x(1))+0.005*(1/lambda)*D1/x(1));
rho_2 = lambda*0.005*(alpha*(N2/x(1))+0.005*(1/lambda)*D2/x(1));
% rho_3 = lambda*K(11,3)*(alpha*(N3/x(1))+(1/lambda)*D3/x(1));
% rho_4 = lambda*K(11,4)*(alpha*(N4/x(1))+(1/lambda)*D4/x(1));
% rho_5 = lambda*K(11,5)*(alpha*(N5/x(1))+(1/lambda)*D5/x(1));
% rho_6 = lambda*K(11,6)*(alpha*(N6/x(1))+(1/lambda)*D6/x(1));
% rho_7 = lambda*K(11,7)*(alpha*(N7/x(1))+(1/lambda)*D7/x(1));
% rho_8 = lambda*K(11,8)*(alpha*(N8/x(1))+(1/lambda)*D8/x(1));
% rho_9 = lambda*K(11,9)*(alpha*(N9/x(1))+(1/lambda)*D9/x(1));
% rho_10 = lambda*K(11,10)*(alpha*(N10/x(1))+(1/lambda)*D10/x(1));
% % rho_11 = lambda*K(11,11)*(alpha*(N11/x(1))+(1/lambda)*D11/x(1));
% rho_12 = lambda*K(11,12)*(alpha*(N12/x(1))+(1/lambda)*D12/x(1));
% 
% %Total reactivity
% 
% rho_t=rho_temp+rho_1+rho_2+rho_3+rho_4+rho_5+rho_6+rho_7+rho_8+rho_9+rho_10+rho_12;

%Reactor Point Kinetics State Equation
rho_t=rho_temp+rho_1+rho_2;

A = [(rho_t-Beta)/lambda L1/lambda L2/lambda;...
    B1 -L1 0;...
    B2 0 -L2];

C = [1 0 0;...
    0 L1 L2];

xdot = zeros(3,1,'double');
xdot = A*x;
y = zeros(2,1,'double');
y = C*x;

return

== matlab function SpatialKineticsOffline/MATLAB Function ==
  data: x input; xdot output; mdoth1 input; mdoth2 input; mdoth3 input; mdoth4 input; mdotc1 input; mdotc2 input; mdotc3 input; mdotc4 input; rxtempout output; Rxtemp1 input; rxwalltempout output; braytontempout output; thirdloopwalltemp output; coolingtowertempout output; Rxtemp2 input; Rxtemp3 input; Rxtemp4 input; Braytonsalt1 input; Braytonsalt2 input; Braytonsalt3 input; Coolingtower input; salttemp output
function [xdot,rxtempout,rxwalltempout,braytontempout,thirdloopwalltemp,coolingtowertempout,salttemp] = ExpandedSaltVault(x,mdoth1,mdoth2,mdoth3,mdoth4,mdotc1,mdotc2,mdotc3,mdotc4,Rxtemp1,Rxtemp2,Rxtemp3,Rxtemp4,Braytonsalt1,Braytonsalt2,Braytonsalt3,Coolingtower)

%%%%% Heat Transfer (HX) coefficients for convention
hr1=3400*7; % HX coefficient for reactor 1
hr2=hr1;    % HX coefficient for reactor 2
hr3=hr1;    % HX coefficient for reactor 3
hr4=hr1;    % HX coefficient for reactor 4
hb1=1000*3; % HX coefficient for Brayton cycle 1
hb2=hb1;    % HX coefficient for Brayton cycle 2
hb3=hb1;    % HX coefficient for Brayton cycle 3
hct=3000;   % HX coefficient for cooling tower 1
hamb=hr1;     % HX coefficient for ambient conditions


%%%%% Mass for different components
mr1=3055;   % mass for reactor 1
mr2=mr1;    % mass for reactor 2
mr3=mr1;    % mass for reactor 3
mr4=mr1;    % mass for reactor 4
ms=60000;   % mass for salt vault
mb1=40*1.5127;  % mass for Brayton cycle 1
mb2=mb1;        % mass for Brayton cycle 2
mb3=mb1;        % mass for Brayton cycle 3
% mct=2000;       % mass for cooling tower 1
mct=500;       % mass for cooling tower 1
Vwall = 0.4675;
rho_tube = 8860;
mrw1 = rho_tube*Vwall;    % mass for wall reactor 1
mrw2 = rho_tube*Vwall;    % mass for wall reactor 2
mrw3 = rho_tube*Vwall;    % mass for wall reactor 3
mrw4 = rho_tube*Vwall;    % mass for wall reactor 4
mbw1 = rho_tube*Vwall;    % mass for wall brayton cycle 1
mbw2 = rho_tube*Vwall;    % mass for wall brayton cycle 2
mbw3 = rho_tube*Vwall;    % mass for wall brayton cycle 3
mctw = rho_tube*Vwall;    % mass for wall cooling tower

%%%%% Specific Heat coefficients
cr1=1901;   % Specific heat for reactor 1
cr2=cr1;    % Specific heat for reactor 2
cr3=cr1;    % Specific heat for reactor 3
cr4=cr1;    % Specific heat for reactor 4
cs=1901;    % Specific heat for salt vault
cb1=965;    % Specific heat for Brayton Cycle 1
cb2=cb1;    % Specific heat for Brayton Cycle 2
cb3=cb1;    % Specific heat for Brayton Cycle 3
cct=5e3;   % Specific heat for cooling tower 1
crw1 = 578; % Specific heat for wall reactor 1
crw2 = 578; % Specific heat for wall reactor 2
crw3 = 578; % Specific heat for wall reactor 3
crw4 = 578; % Specific heat for wall reactor 4
cbw1 = 578; % Specific heat for wall brayton cycle 1
cbw2 = 578; % Specific heat for wall brayton cycle 2
cbw3 = 578; % Specific heat for wall brayton cycle 3
cctw = 578; % Specific heat for wall cooling tower

%%%%% Area for different components
Ar1=292;    % Area for reactor 1
Ar2=Ar1;    % Area for reactor 2
Ar3=Ar1;    % Area for reactor 3
Ar4=Ar1;    % Area for reactor 4
Ab1=Ar1;    % Area for Brayton cycle 1
Ab2=Ar1;    % Area for Brayton cycle 2
Ab3=Ar1;    % Area for Brayton cycle 3
Act=Ar1;    % Area for cooling tower
Asurface=2000*pi(); % Area 

%%%%% Mass Flow Rates
% mdoth1 = mdotinput(1);
% mdoth2 = mdotinput(2);
% mdoth3 = mdotinput(3);
% mdoth4 = mdotinput(4);
% mdotc1 = mdotinput(5);
% mdotc2 = mdotinput(6);
% mdotc3 = mdotinput(7);
% mdotc4 = mdotinput(8);


%%%%% State-Space Representation

%%% State matrix
A = zeros(17,17);
A(1,(1:2)) = [-(mdoth1*cr1+hr1*Ar1)/(mr1*cr1) hr1*Ar1/(mr1*cr1)];
A(2, [1 2 17]) = [Ar1*hr1/(mrw1*crw1) -(Ar1*hr1+Ar1*hamb)/(mrw1*crw1) Ar1*hamb/(mrw1*crw1)];
A(3,(3:4)) = [-(mdoth2*cr2+hr2*Ar2)/(mr2*cr2) hr2*Ar2/(mr2*cr2)];
A(4, [3 4 17]) = [Ar2*hr2/(mrw2*crw2) -(Ar2*hr2+Ar2*hamb)/(mrw2*crw2) Ar2*hamb/(mrw2*crw2)];
A(5,(5:6)) = [-(mdoth3*cr3+hr3*Ar3)/(mr3*cr3) hr3*Ar3/(mr3*cr3)];
A(6, [5 6 17]) = [Ar3*hr3/(mrw3*crw3) -(Ar3*hr3+Ar3*hamb)/(mrw3*crw3) Ar3*hamb/(mrw3*crw3)];
A(7,(7:8)) = [-(mdoth4*cr4+hr4*Ar4)/(mr4*cr4) hr4*Ar4/(mr4*cr4)];
A(8, [7 8 17]) = [Ar4*hr4/(mrw4*crw4) -(Ar4*hr4+Ar4*hamb)/(mrw4*crw4) Ar4*hamb/(mrw4*crw4)];
A(9,(9:10)) = [-(mdotc1*cb1+hb1*Ab1)/(mb1*cb1) hb1*Ab1/(mb1*cb1)];
A(10, [9 10 17]) = [Ab1*hb1/(mbw1*cbw1) -(Ab1*hb1+Ab1*hamb)/(mbw1*cbw1) Ab1*hamb/(mbw1*cbw1)];
A(11,(11:12)) = [-(mdotc2*cb2+hb2*Ab2)/(mb2*cb2) hb2*Ab2/(mb2*cb2)];
A(12, [11 12 17]) = [Ab2*hb2/(mbw2*cbw2) -(Ab2*hb2+Ab2*hamb)/(mbw2*cbw2) Ab2*hamb/(mbw2*cbw2)];
A(13,(13:14)) = [-(mdotc3*cb3+hb3*Ab3)/(mb3*cb3) hb3*Ab3/(mb3*cb3)];
A(14, [13 14 17]) = [Ab3*hb3/(mbw3*cbw3) -(Ab3*hb3+Ab3*hamb)/(mbw3*cbw3) Ab3*hamb/(mbw3*cbw3)];
A(15,(15:16)) = [-(mdotc4*cct+hct*Act)/(mct*cct) hct*Act/(mct*cct)];
A(16, [15 16 17]) = [Act*hct/(mctw*cctw) -(Act*hct+Act*hamb)/(mctw*cctw) Act*hamb/(mctw*cctw)];
A(17,[2:2:16 17]) = [Ar1*hamb/(ms*cs) Ar2*hamb/(ms*cs) Ar3*hamb/(ms*cs) Ar4*hamb/(ms*cs) Ab1*hamb/(ms*cs) Ab2*hamb/(ms*cs) Ab3*hamb/(ms*cs) Act*hamb/(ms*cs) -(Ar1*hamb + Ab1*hamb + Ar2*hamb + Ab2*hamb + Ar3*hamb + Ab3*hamb + Ar4*hamb + Act*hamb)/(ms*cs)];

%%% Input matrix Inlet Temperature
Btemp = zeros(17,8);
Btemp(1,1) = mdoth1/mr1;
Btemp(3,2) = mdoth2/mr2;
Btemp(5,3) = mdoth3/mr3;
Btemp(7,4) = mdoth4/mr4;
Btemp(9,5) = mdotc1/mb1;
Btemp(11,6) = mdotc2/mb2;
Btemp(13,7) = mdotc3/mb3;
Btemp(15,8) = mdotc4/mct;

%%% Output Matrix
C = eye(17);

%%% State-space equations
tempinput = [Rxtemp1,Rxtemp2,Rxtemp3,Rxtemp4,Braytonsalt1,Braytonsalt2,Braytonsalt3,Coolingtower]';
xdot = A*x + Btemp*tempinput;
y = C*x;
rxtempout = y([1 3 5 7],1);
rxwalltempout = y([2:2:8],1);
braytontempout = y([9:2:13],1);
thirdloopwalltemp = y([10:2:16],1);
coolingtowertempout = y(15,1);
salttemp = y(17,1);



return
